simulink model "untitled"  (R2023b)
settings: Solver=VariableStepAuto  StartTime=0.0  StopTime=10.0  RelTol=1e-3
libraries: dspsrcs4 x1
settings Model: Creator=maxim  LastModifiedBy=maxim

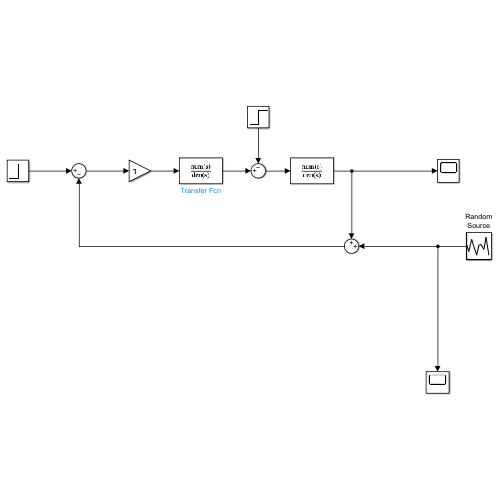
[thumbnail: Simulink's stored preview of the top-level diagram]
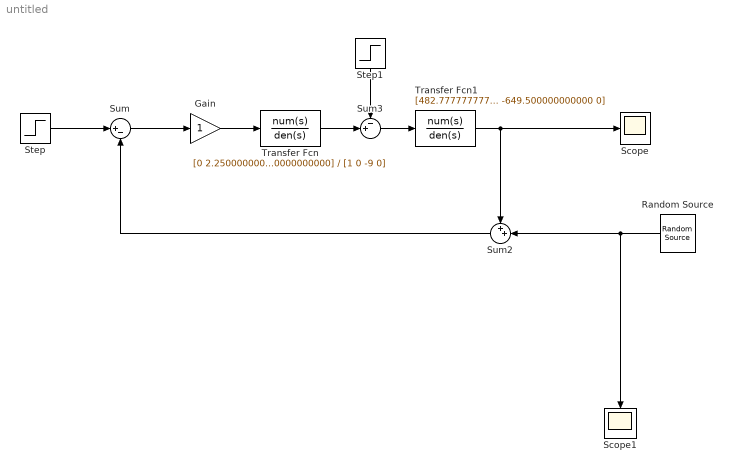
== system untitled ==
  Gain : Gain
  Random Source : dspsrcs4/Random Source  SrcType=Gaussian  NormMethod=Ziggurat  CltLength=12  MinVal=0  MaxVal=1  MeanVal=0  VarVal=0.1  RepMode=Not repeatable  rawSeed=1  IsInherit=off  SampMode=Discrete  SampTime=1/100  SampFrame=1  DataType=Double  OutComplex=Real  OutputFrames=off
  Scope : Scope
  Scope1 : Scope
  Step : Step  After=20  SampleTime=0
  Step1 : Step  Time=1.1  SampleTime=0
  Sum : Sum  Inputs=|+-
  Sum2 : Sum  Inputs=++|
  Sum3 : Sum  Inputs=-+|
  Transfer Fcn : TransferFcn  Numerator=[0 2.25000000000000 -2.25000000000000 -4.50000000000000]  Denominator=[1 0 -9 0]
  Transfer Fcn1 : TransferFcn  Numerator=[482.777777777778 935 -1502.22222222222 0]  Denominator=[1 -1052.25000000000 -649.500000000000 0]
  wires:
  Step/1 -> Sum/1
  Step1/1 -> Sum3/1
  Sum2/1 -> Sum/2
  Sum/1 -> Gain/1
  Gain/1 -> Transfer Fcn/1
  Random Source/1 -> Scope1/1, Sum2/2
  Sum3/1 -> Transfer Fcn1/1
  Transfer Fcn/1 -> Sum3/2
  Transfer Fcn1/1 -> Scope/1, Sum2/1
